simulink model "model_bo"  (Simulink 4.00)
settings: Solver=ode45  StartTime=0.0  StopTime=10.0  RelTol=1e-3
undefined symbols (not defined in the file): a1_A5, a2_A5, A_B1, B_B1, C_B1, D_B1, den_pade_A1, den_pade_A5, num_pade_A1, num_pade_A5
settings Model: Creator=fromion  LastModifiedBy=administrateur  LimitDataPoints=off  ExtModeTrigMode=oneshot  ExtModeArmWhenConnect=off

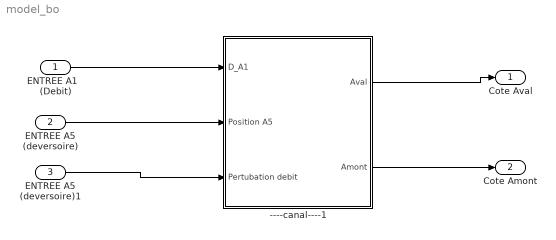
== system model_bo ==
  ENTREE A1   (Debit) : Inport  Port=1  LatchInput=off
  ENTREE A5 (deversoire) : Inport  Port=2  LatchInput=off
  ENTREE A5 (deversoire)1 : Inport  Port=3  LatchInput=off
  ----canal----1 : Subsystem
      settings: RTWFcnNameOpts=Auto  RTWFileNameOpts=Auto
  Cote Aval : Outport  Port=1
  "Cote Amont " : Outport  Port=2
  wires:
  ----canal----1/1(Aval) -> Cote Aval/1
  ----canal----1/2(Amont) -> "Cote Amont "/1
  ENTREE A1   (Debit)/1 -> ----canal----1/1("D_A1 ")
  ENTREE A5 (deversoire)/1 -> ----canal----1/2(Position A5)
  ENTREE A5 (deversoire)1/1 -> ----canal----1/3(Pertubation debit)

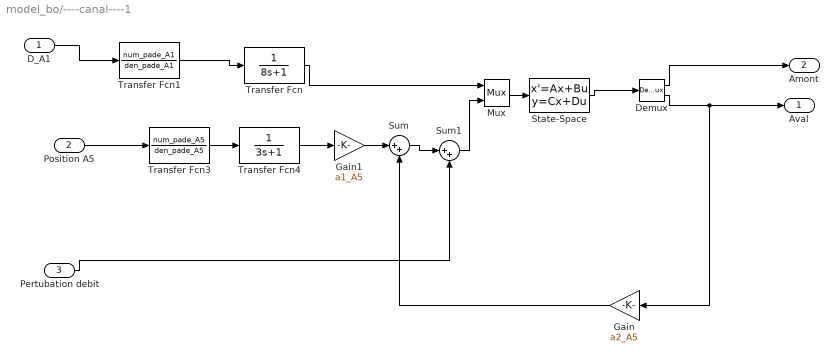
== system model_bo/----canal----1 ==
  "D_A1 " : Inport  Port=1  LatchInput=off
  Position A5 : Inport  Port=2  LatchInput=off
  Pertubation debit : Inport  Port=3  LatchInput=off
  Demux : Demux  Outputs=2  BusSelectionMode=off
  Gain : Gain  Orientation=left  Gain=a2_A5  Multiplication=Element-wise(K.*u)  SaturateOnIntegerOverflow=on
  Gain1 : Gain  Gain=a1_A5  Multiplication=Element-wise(K.*u)  SaturateOnIntegerOverflow=on
  Mux : Mux  Inputs=2
      settings: DisplayOption=none
  State-Space : StateSpace  A=A_B1  B=B_B1  C=C_B1  D=D_B1  X0=0  AbsoluteTolerance=auto  Realization=auto
  Sum : Sum  Inputs=|++  SaturateOnIntegerOverflow=on
  Sum1 : Sum  Inputs=|++  SaturateOnIntegerOverflow=on
  Transfer Fcn : TransferFcn  Numerator=[1]  Denominator=[8 1]  AbsoluteTolerance=auto  Realization=auto
  Transfer Fcn1 : TransferFcn  Numerator=num_pade_A1  Denominator=den_pade_A1  AbsoluteTolerance=auto  Realization=auto
  Transfer Fcn3 : TransferFcn  Numerator=num_pade_A5  Denominator=den_pade_A5  AbsoluteTolerance=auto  Realization=auto
  Transfer Fcn4 : TransferFcn  Numerator=[1]  Denominator=[3 1]  AbsoluteTolerance=auto  Realization=auto
  Aval : Outport  Port=1
  Amont : Outport  Port=2
  wires:
  Mux/1 -> State-Space/1
  State-Space/1 -> Demux/1
  Demux/2 -> Aval/1, Gain/1
  Demux/1 -> Amont/1
  Gain/1 -> Sum/2
  Transfer Fcn3/1 -> Transfer Fcn4/1
  Position A5/1 -> Transfer Fcn3/1
  Transfer Fcn1/1 -> Transfer Fcn/1
  Transfer Fcn/1 -> Mux/1
  "D_A1 "/1 -> Transfer Fcn1/1
  Transfer Fcn4/1 -> Gain1/1
  Gain1/1 -> Sum/1
  Sum/1 -> Sum1/1
  Sum1/1 -> Mux/2
  Pertubation debit/1 -> Sum1/2
